simulink model "pr434"  (R2018b)
settings: Solver=VariableStepAuto  StartTime=0.0  StopTime=inf  RelTol=1e-3  EnableMultiTasking=on
PreLoadFcn:
  | pr434setup; % скрипт инициализации параметров
values from neighbouring files (symbols this model uses):
  beta = 0.2    [pr434setup.m]
  fc = 10e6    (= 10000000)    [pr434setup.m]
  fs = rsym * nsamp    (= 50000000)    [pr434setup.m]
  M = 4    [pr434setup.m]
  nsamp = 50    [pr434setup.m]
  nsym = 8    [pr434setup.m]
  rsym = 1e6    (= 1000000)    [pr434setup.m]
libraries: dspsrcs4 x3, commfilt2 x2, commdigbbndam3 x2, commutil2 x1, commchan3 x1, commrandsrc3 x1, dsparch4 x1, commsink2 x1, commrflib2 x1
CloseFcn:
  | clear all;
settings Model: Creator=GRIHA  LastModifiedBy=Григорий Фокин
settings DataIOCC: LimitDataPoints=on
settings OptimizationCC: LifeSpan=inf
settings DebuggingCC: AllowSymbolicDim=off  SFUnexpectedBacktrackingDiag=warning  SFNoUnconditionalDefaultTransitionDiag=warning  SFExecutionAtInitializationDiag=none
settings ModelReferenceCC: PropagateSignalLabelsOutOfModel=off
settings SFSimCC: SimUseLocalCustomCode=off
settings RTWCC: RTWUseLocalCustomCode=off
settings CodeAppCC: StateflowObjectComments=on
settings GRTTargetCC: TargetLangStandard=C89/C90 (ANSI)
settings ConfigComp: CovMetricSettings=dw  CovHtmlReporting=on  CovSaveCumulativeToWorkspaceVar=on  CovSaveSingleToWorkspaceVar=on  CovExternalEMLEnable=off

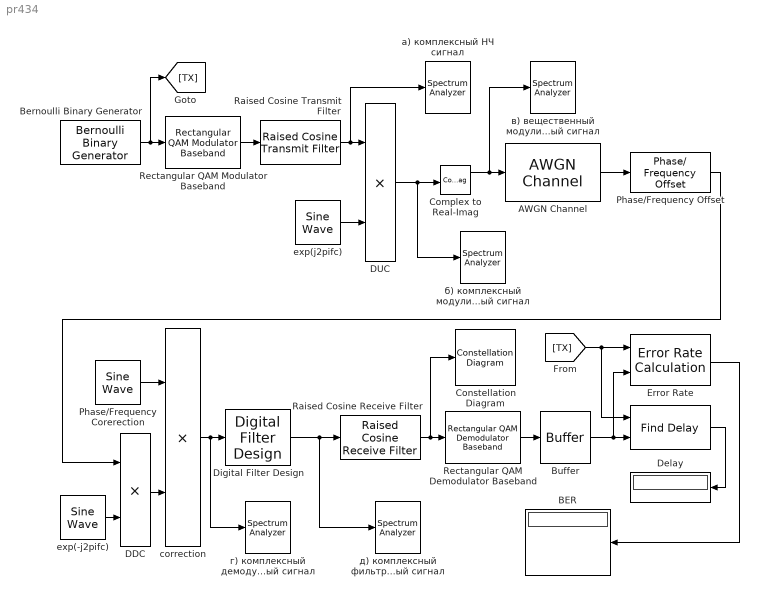
== system pr434 ==
  " " : commutil2/Find Delay  corrLength=1000  chgSigOP=off  stopUpdate=off  numConstDelay=3
      settings: SourceProductName=Communications System Toolbox  SourceProductBaseCode=CM
  AWGN Channel : commchan3/AWGN Channel  InputProcessing=Columns as channels (frame based)  seed=67  noiseMode="Signal to noise ratio  (SNR)"  EbNodB=10  EsNodB=10  SNRdB=SNR  bitsPerSym=1  Ps=sigpower  Tsym=1  variance=1
  BER : Display
  Bernoulli Binary Generator : commrandsrc3/Bernoulli Binary Generator  ProbabilityOfZero=0.5  SeedSource=Auto  Seed=0  SampleTime=1/rsym/log2(M)  SamplesPerFrame=log2(M)  OutputDataType=double  SimulateUsing=Interpreted execution
  Buffer : Buffer  N=log2(M)  OutputFrames=off
  Complex to Real-Imag : ComplexToRealImag
  Constellation Diagram : ConstellationDiagram
  DDC : Product
  DUC : Product
  Delay : Display
  Digital Filter Design : dsparch4/Digital Filter Design  mwdsp_browser_bugfix_var=off
  Error Rate : commsink2/Error Rate Calculation  N=22  st_delay=0  cp_mode=Entire frame  subframe=[]  PMode=Port  WsName=ErrorVec  RsMode2=off  stop=off  numErr=100  maxBits=1e6
  Phase/Frequency Corerection : dspsrcs4/Sine Wave  Amplitude=1  Frequency=0  Phase=-pi/4  SampleMode=Discrete  OutComplex=Complex  CompMethod=Trigonometric fcn  TableSize=Speed  SampleTime=1/fs  SamplesPerFrame=1  ResetState=Restart at time zero  OutputFrames=off  dataType=double  wordLen=16  udDataType=sfix(16)  fracBitsMode=Best precision  numFracBits=15  OutDataTypeStr=double  LastOutDataTypeStr=double
  Phase/Frequency Offset : commrflib2/Phase// Frequency Offset  phaseOffset=45  freqPort=off  freqOffset=0
      settings: SourceProductName=Communications System Toolbox
  Raised Cosine Receive Filter : commfilt2/Raised Cosine Receive Filter  filtType=Square root  R=beta  filtSpan=nsym  N=nsamp  downFactor=nsamp  downOffset=0  filterGain=1  RateOptions=Allow multirate processing  framing=Mute  checkCoeff=off  variableName=rcRxFilt1  currentFiltSpan=nsym  D=(nsym)/2  inputOffset=0  sampMode=Mute  saveAsFlag=0  rateMode=Downsampling  checkGain=Normalized  launchFVT=on  roundingMode=Floor  overflowMode=off  coeffDataTypeStr=Inherit: Same word length as input  coeffMin=[]  coeffMax=[]  coeffLastDataTypeStr=Inherit: Same word length as input  accumDataTypeStr=Inherit: Same as product output  accumLastDataTypeStr=Inherit: Same as product output  outputDataTypeStr=Inherit: Same as accumulator  outputMin=[]  outputMax=[]  outputLastDataTypeStr=Inherit: Same as accumulator
  Raised Cosine Transmit Filter : commfilt2/Raised Cosine Transmit Filter  filtType=Square root  R=beta  filtSpan=nsym  N=nsamp  filterGain=1  RateOptions=Allow multirate processing  framing=Mute  checkCoeff=on  variableName=rcTxFilt  checkGain=Normalized  sampMode=Mute  saveAsFlag=0  currentFiltSpan=nsym  D=(nsym)/2  launchFVT=on  roundingMode=Floor  overflowMode=off  coeffDataTypeStr=Inherit: Same word length as input  coeffMin=[]  coeffMax=[]  coeffLastDataTypeStr=Inherit: Same word length as input  outputDataTypeStr=Inherit: Same as accumulator  outputMin=[]  outputMax=[]  outputLastDataTypeStr=Inherit: Same as accumulator
  Rectangular QAM Demodulator Baseband : commdigbbndam3/Rectangular QAM Demodulator Baseband  M=M  OutType=Bit  DecType=Hard decision  VarSource=Dialog  Variance=1  Dec=Gray  Mapping=[0:15]  PowType=Min. distance between symbols  MinDist=2  AvgPow=1  PeakPow=1  Ph=0  outDtype1=Inherit via internal rule  outDtype2=Inherit via internal rule  derotateFactorWordLen=16  derotateFactorDataTypeStr=Inherit: Same word length as input  derotateFactorLastDataTypeStr=Inherit: Same word length as input  denormFactorWordLen=16  denormFactorDataTypeStr=Inherit: Same word length as input  denormFactorLastDataTypeStr=Inherit: Same word length as input  prodOutWordLen=32  prodOutOverflowMode=Wrap  prodOutRoundingMode=Floor  prodOutOvFlMode=off  prodOutOvFlModeLastStrValue=off  sumWordLen=32
  Rectangular QAM Modulator Baseband : commdigbbndam3/Rectangular QAM Modulator Baseband  M=M  InType=Bit  Enc=Gray  Mapping=[0:15]  PowType=Min. distance between symbols  MinDist=2  AvgPow=1  PeakPow=1  Ph=0  outDtype=double  outWordLen=16  outUDDataType=sfix(16)  outFracLenMode=Best precision  outFracLen=15  outDataTypeStr=double  outLastDataTypeStr=double
  correction : Product
  exp(-j2pifc) : dspsrcs4/Sine Wave  Amplitude=1  Frequency=-fc  Phase=0  SampleMode=Discrete  OutComplex=Complex  CompMethod=Trigonometric fcn  TableSize=Speed  SampleTime=1/fs  SamplesPerFrame=1  ResetState=Restart at time zero  OutputFrames=off  dataType=double  wordLen=16  udDataType=sfix(16)  fracBitsMode=Best precision  numFracBits=15  OutDataTypeStr=double  LastOutDataTypeStr=double
  exp(j2pifc) : dspsrcs4/Sine Wave  Amplitude=1  Frequency=fc  Phase=0  SampleMode=Discrete  OutComplex=Complex  CompMethod=Trigonometric fcn  TableSize=Speed  SampleTime=1/fs  SamplesPerFrame=1  ResetState=Restart at time zero  OutputFrames=off  dataType=double  wordLen=16  udDataType=sfix(16)  fracBitsMode=Best precision  numFracBits=15  OutDataTypeStr=double  LastOutDataTypeStr=double
  а) комплексный НЧ сигнал : SpectrumAnalyzer
  б) комплексный модулированный сигнал : SpectrumAnalyzer
  в) вещественный модулированный сигнал : SpectrumAnalyzer
  г) комплексный демодулированный сигнал : SpectrumAnalyzer
  д) комплексный фильтрованный сигнал : SpectrumAnalyzer
  wires:
  Bernoulli Binary Generator/1 -> Rectangular QAM Modulator Baseband/1, [TX]
  Rectangular QAM Modulator Baseband/1 -> Raised Cosine Transmit Filter/1
  DUC/1 -> Complex to Real-Imag/1, б) комплексный модулированный сигнал/1
  exp(j2pifc)/1 -> DUC/2
  Raised Cosine Transmit Filter/1 -> а) комплексный НЧ сигнал/1, DUC/1
  Complex to Real-Imag/1 -> AWGN Channel/1, в) вещественный модулированный сигнал/1
  AWGN Channel/1 -> Phase/Frequency Offset/1
  Phase/Frequency Offset/1 -> DDC/1
  exp(-j2pifc)/1 -> DDC/2
  Rectangular QAM Demodulator Baseband/1 -> Buffer/1
  " "/1 -> Delay/1
  [TX] -> Error Rate/1, " "/1
  Error Rate/1 -> BER/1
  Raised Cosine Receive Filter/1 -> Rectangular QAM Demodulator Baseband/1, Constellation Diagram/1
  Digital Filter Design/1 -> Raised Cosine Receive Filter/1, д) комплексный фильтрованный сигнал/1
  DDC/1 -> correction/2
  correction/1 -> г) комплексный демодулированный сигнал/1, Digital Filter Design/1
  Phase/Frequency Corerection/1 -> correction/1
  Buffer/1 -> Error Rate/2, " "/2
